simulink model "lab3_model_2"  (R2015a)
settings: Solver=ode3  SolverMode=SingleTasking  StartTime=0.0  StopTime=10.0  FixedStep=1e-2  RelTol=1e-2
values from neighbouring files (symbols this model uses):
  A = [ -2  0 ... (first row only)    [script.m]    (also in script1.m = 1; script2.m = Ap; script3.m = [0 1;-5 -8])
  AP = expm(A*h)    [script3.m]
  B = [ -1 ... (first row only)    [script.m]    (also in script2.m = Bp; script3.m = [0;1])
  BP = double( int(expm(x*A)*B,x,0,h))    [script3.m]
  C = [ 1.5 0.2 ]    [script.m]    (also in script2.m = eye(2); script3.m = eye(2))
  CP = C    [script3.m]
  freq = .1    (= 0.1)    [script3.m]
  h = 3    [script.m]    (also in script2.m = 0.5; script3.m = h+i/5)
  WPC = 1    [script2.m]    (also in script3.m = 0)
settings Model: Creator=bb  LastModifiedBy=bb

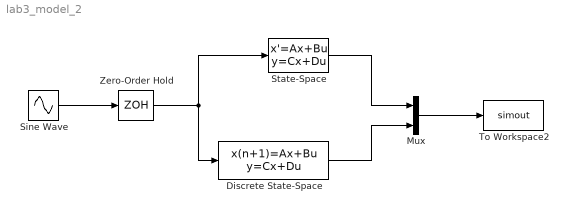
== system lab3_model_2 ==
  Discrete State-Space : DiscreteStateSpace  A=AP  B=BP  C=CP  D=[0;0]  X0=WPC  SampleTime=h
  Mux : Mux  Inputs=2
  Sine Wave : Sin  Frequency=freq  SampleTime=0
  State-Space : StateSpace  A=A  B=B  C=C  D=[0;0]  X0=WPC
  To Workspace2 : ToWorkspace  VariableName=simout  SampleTime=-1
  Zero-Order Hold : ZeroOrderHold  SampleTime=h
  wires:
  Zero-Order Hold/1 -> State-Space/1, Discrete State-Space/1
  Sine Wave/1 -> Zero-Order Hold/1
  State-Space/1 -> Mux/1
  Discrete State-Space/1 -> Mux/2
  Mux/1 -> To Workspace2/1
